simulink model "brushed_dc_motor_pi_velocity"  (R2024a)
settings: Solver=VariableStepAuto  StartTime=0.0  StopTime=10.0  RelTol=1e-3
values from neighbouring files (symbols this model uses):
  c = 10e-4    (= 0.001)    [brushed_dc_motor_PID_example1.m]    (also in brushed_dc_motor_PID_example2.m; brushed_dc_motor_PID_example3.m; brushed_dc_motor_example1.m)
  I = 9e-5    (= 9e-05)    [brushed_dc_motor_PID_example1.m]    (also in brushed_dc_motor_PID_example2.m; brushed_dc_motor_PID_example3.m; brushed_dc_motor_example1.m)
  Kb = Kt    (= 0.05)    [brushed_dc_motor_PID_example1.m]    (also in brushed_dc_motor_PID_example2.m; brushed_dc_motor_PID_example3.m; brushed_dc_motor_example1.m)
  Ki = 50    [brushed_dc_motor_PID_example2.m]    (also in brushed_dc_motor_PID_example3.m)
  Kp = 1000    [brushed_dc_motor_PID_example1.m]    (also in brushed_dc_motor_PID_example2.m = 100; brushed_dc_motor_PID_example3.m = 100)
  Kt = 0.05    [brushed_dc_motor_PID_example1.m]    (also in brushed_dc_motor_PID_example2.m; brushed_dc_motor_PID_example3.m; brushed_dc_motor_example1.m)
  La = 2e-3    (= 0.002)    [brushed_dc_motor_PID_example1.m]    (also in brushed_dc_motor_PID_example2.m; brushed_dc_motor_PID_example3.m; brushed_dc_motor_example1.m)
  Ra = 0.5    [brushed_dc_motor_PID_example1.m]    (also in brushed_dc_motor_PID_example2.m; brushed_dc_motor_PID_example3.m; brushed_dc_motor_example1.m)
  Tl = 1    [brushed_dc_motor_PID_example1.m]    (also in brushed_dc_motor_PID_example2.m = 3; brushed_dc_motor_PID_example3.m = 3; brushed_dc_motor_example1.m)
  wref = 10    [brushed_dc_motor_PID_example1.m]    (also in brushed_dc_motor_PID_example2.m; brushed_dc_motor_PID_example3.m)
settings Model: Creator=thill  LastModifiedBy=thill

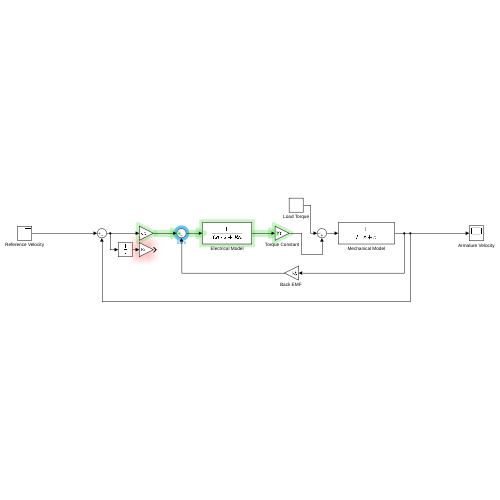
[thumbnail: Simulink's stored preview of the top-level diagram]
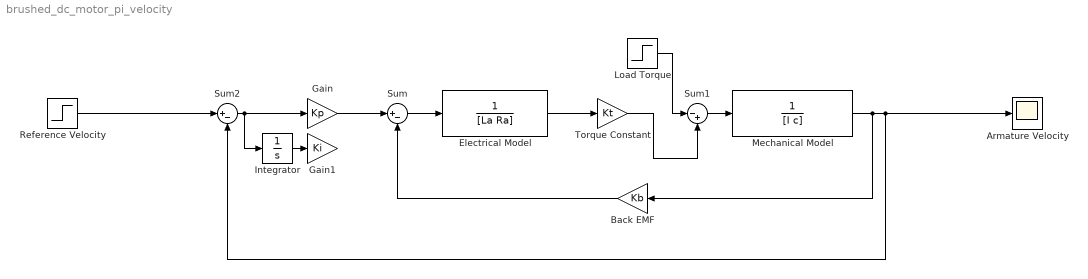
== system brushed_dc_motor_pi_velocity ==
  Armature Velocity : Scope
  "Back EMF " : Gain  Gain=Kb
  Electrical Model : TransferFcn  Denominator=[La Ra]
  Gain : Gain  Gain=Kp
  Gain1 : Gain  Gain=Ki
  Integrator : Integrator
  Load Torque : Step  After=Tl  SampleTime=0
  Mechanical Model : TransferFcn  Denominator=[I c]
  Reference Velocity : Step  After=wref  SampleTime=0
  Sum : Sum  Inputs=|+-
  Sum1 : Sum  Inputs=|-+
  Sum2 : Sum  Inputs=|+-
  Torque Constant : Gain  Gain=Kt
  wires:
  Sum/1 -> Electrical Model/1
  "Back EMF "/1 -> Sum/2
  Sum1/1 -> Mechanical Model/1
  Load Torque/1 -> Sum1/1
  Torque Constant/1 -> Sum1/2
  Electrical Model/1 -> Torque Constant/1
  Sum2/1 -> Integrator/1, Gain/1
  Gain/1 -> Sum/1
  Reference Velocity/1 -> Sum2/1
  Mechanical Model/1 -> Armature Velocity/1, Sum2/2, "Back EMF "/1
  Integrator/1 -> Gain1/1
